simulink model "FurutaStateSpace"  (R2025b)
settings: Solver=FixedStepAuto  StartTime=0.0  StopTime=10  FixedStep=0.001  RelTol=1e-3
settings Model: Creator=kingb  LastModifiedBy=kingb

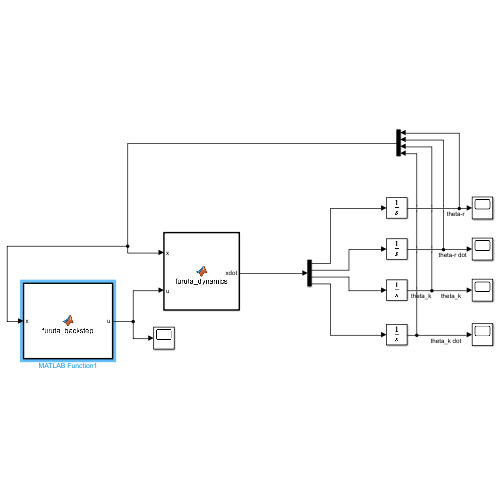
[thumbnail: Simulink's stored preview of the top-level diagram]
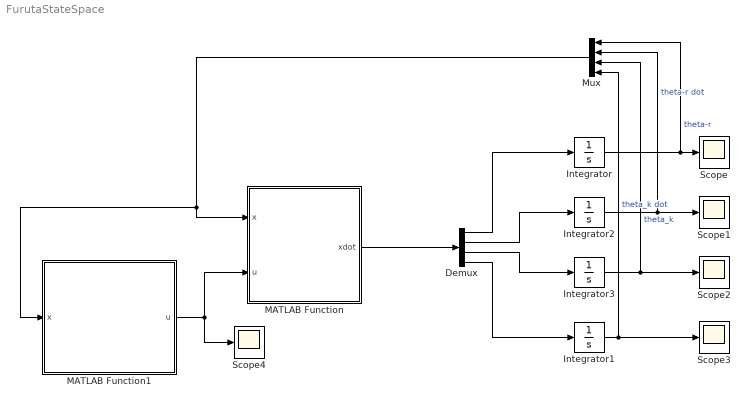
== system FurutaStateSpace ==
  Demux : Demux
  Integrator{,1..3} (4 alike) : Integrator
  MATLAB Function : MATLAB Function  TreatAsAtomicUnit=on
  MATLAB Function1 : MATLAB Function  TreatAsAtomicUnit=on
  Mux : Mux
  Scope{,1..4} (5 alike) : Scope
      Scope settings: ActiveDisplayYMinimum=-28.978126511604493  ActiveDisplayYMaximum=79.46073870424118
      Scope1 settings: ActiveDisplayYMinimum=-1  ActiveDisplayYMaximum=1
      Scope2 settings: ActiveDisplayYMinimum=2.7844311487267892  ActiveDisplayYMaximum=3.389538393974846  DataLoggingVariableName=ScopeData2
      Scope3 settings: ActiveDisplayYMinimum=-1  ActiveDisplayYMaximum=1  DataLoggingVariableName=ScopeData3
      Scope4 settings: ActiveDisplayYMinimum=-0.99292213805658158  ActiveDisplayYMaximum=1.4363799000726727  DataLoggingVariableName=ScopeData4
  wires:
  Integrator1/1 -> Mux/4, Scope3/1  "theta_k dot"
  Integrator3/1 -> Mux/3, Scope2/1  "theta_k"
  Integrator2/1 -> Mux/2, Scope1/1  "theta-r dot"
  Integrator/1 -> Mux/1, Scope/1  "theta-r"
  Mux/1 -> MATLAB Function1/1(x), MATLAB Function/1(x)
  MATLAB Function1/1(u) -> MATLAB Function/2(u), Scope4/1
  MATLAB Function/1(xdot) -> Demux/1
  Demux/2 -> Integrator2/1
  Demux/3 -> Integrator3/1
  Demux/1 -> Integrator/1
  Demux/4 -> Integrator1/1

== matlab function FurutaStateSpace/MATLAB Function1 ==
  settings: updateMethod=DISCRETE
  data: x input size=4; u output
function u = furuta_backstep(x)
    % State vector: x = [theta_r; dtheta_r; theta_k; dtheta_k]
    theta_r = x(1);  
    dtheta_r = x(2);
    theta_k = x(3);  
    dtheta_k = x(4);

    % Physical parameters (as given)
    mk = 0.15;  
    lk = 0.20;  
    lr = 0.20;
    Ik = 0.004;  
    Ir = 0.006;  
    g = 9.81;
    Bk = 0.0008;  
    Br = 0.002;

    %_______________________SYSTEM DYNAMICS__________________________

    % --- Mass/Inertia matrix ---
    M11 = Ir + mk*lr^2 + mk*lk^2*sin(theta_k)^2;
    M12 = mk*lr*lk*cos(theta_k);
    M21 = M12;
    M22 = Ik + mk*lk^2;

    % --- Coriolis/centrifugal terms ---
    C1 = mk*lk^2*sin(theta_k)*cos(theta_k)*dtheta_k^2;

    % --- Damping ---
    F1 = Br*dtheta_r;



    if abs(theta_k) >= pi - 0.8 && abs(theta_k) <= pi + 0.8
    
        %_______________________BACKSTEPPING__________________________
        
        % Gains
        k1 = 30;
        k2 = 15;
        k3 = -21;
    
        % subsystems
    
        z1 = theta_k - pi;          % error from upright
        z1 = mod(z1+pi, 2*pi) - pi; % Wrap error to [-pi,pi] if desired:
    
        z2 = dtheta_k + k1*z1;
    
        z3 = dtheta_r;
  
    
        % pendulum system coeff
    
        a = -(mk *g * lk * sin(theta_k) + Bk * dtheta_k) / M22;
    
        b = -M12 / M22;
    
        % Avoid division by zero in extreme case
        if abs(b) < 1e-6
            b = sign(b)*1e-6;
        end
    
   
        %for the control of the arm velocity
    
        theta_r_doubledot_star = (-k1*dtheta_k - k2*z2 - a)/b;
    
    
        theta_r_doubledot = theta_r_doubledot_star - k3*z3;
    
    
    
        theta_k_doubledot = a + b * theta_r_doubledot;
    
        u = M11*theta_r_doubledot + M12*theta_k_doubledot + C1 + F1;




    else 
    
        %_______________________energy-based swing-up__________________________
    
        % Compute omega_0 
        omega_0 = sqrt(mk * g * lk / Ik); 
        
        % Normalized energy E 
        E = (mk * g * lk / 2) * ((dtheta_k / omega_0)^2 + cos(theta_k) - 1); 
        
        % Desired energy E0 = 0 (upright) 
        
        E0 = 0; 
        
        % Gain kv 
        kv = -1.5; 
        
        %kick start for when pendulum is at the bottom  
        kick = 0; 
        
        if abs(theta_k) < 0.3 
            kick = 1.0 * tanh(5 * (0.3 - abs(theta_k))) * sign(theta_k); %works for all values except -0.1 to -0.8 
                                                         % if u add sign(theta_k) it works for all values except 0 
            if abs(theta_k) < 0.25 && abs(dtheta_k) < 0.2
                  kick = 0.6 * sign(cos(theta_k));  % always pushes forward
            end
        end 
    
        % Sign term for direction 
        sign_term = sign(dtheta_k * cos(theta_k)); 
        
        % Control torque
        
        u = kv * (E - E0) * sign_term + kick; 
    end


    u = max(min(u, 1), -1);
end

== matlab function FurutaStateSpace/MATLAB Function ==
  data: x input; xdot output; u input
function xdot = furuta_dynamics(x, u)

%   x = [theta_r; dtheta_r; theta_k; dtheta_k]
%   theta_r = arm angle (rad)
%   dtheta_r = arm angular velocity (rad/s)
%   theta_k = pendulum angle (rad) from upright vertical
%   dtheta_k = pendulum angular velocity (rad/s)


    % --- states ---
    theta_r  = x(1);
    dtheta_r = x(2);
    theta_k  = x(3);
    dtheta_k = x(4);

    tau = u;


    % --- Physical parameters ---
    mk = 0.15;   % pendulum mass [kg]
    lk = 0.20;   % pendulum length to CoM [m]
    lr = 0.20;   % arm length [m]
    Ik = 0.004;  % pendulum inertia [kg*m^2]
    Ir = 0.006;  % arm inertia [kg*m^2]
    g  = 9.81;   % gravity [m/s^2]
    Bk = 0.0008; % pendulum damping [N*m*s/rad]
    Br = 0.002;  % arm damping [N*m*s/rad]


    % --- Mass/Inertia matrix ---
    M11 = Ir + mk*lr^2 + mk*lk^2*sin(theta_k)^2;
    M12 = mk*lr*lk*cos(theta_k);
    M21 = M12;
    M22 = Ik + mk*lk^2;

    M = [M11, M12; M21, M22];


    % --- Coriolis/centrifugal terms ---
    C1 = mk*lk^2*sin(theta_k)*cos(theta_k)*dtheta_k^2;
    C2 = 0;  % often negligible for single DOF pendulum

    C = [C1; C2];


    % --- Gravity vector ---
    G1 = 0;         % arm is horizontal, gravity does not affect it
    G2 = mk*g*lk*sin(theta_k);

    G = [G1; G2];



    % --- Damping ---
    F = [Br*dtheta_r; Bk*dtheta_k];



    % --- Compute accelerations ---
    % Solve: M*[ddtheta_r; ddtheta_k] = [tau; 0] - C - G - F
    accel = M \ ([tau; 0] - C - G - F);

    ddtheta_r = accel(1);
    ddtheta_k = accel(2);



    % --- State derivative ---
    xdot = [dtheta_r;
            ddtheta_r;
            dtheta_k;
            ddtheta_k];

end
